simulink model "five"  (R2019b)
settings: Solver=VariableStepAuto  StartTime=0.0  StopTime=2  RelTol=1e-3
undefined symbols (not defined in the file): magnitude
libraries: dsparch4 x2, commsynccomp2 x1
settings Model: Creator=Lenovo  LastModifiedBy=Lenovo

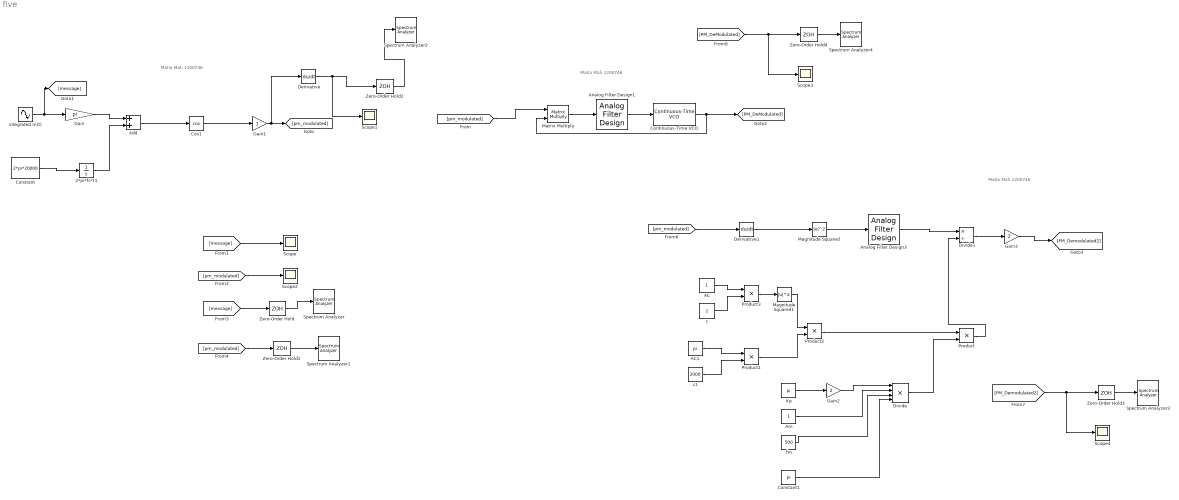
== system five ==
  note: Maha Mali 1200746
  note: Maha Mali 1200746
  note: Maha Mali 1200746
  2*pi*fc*t1 : Integrator
  AC : Constant
  AC1 : Constant  Value=pi
  Add : Sum
  Am : Constant
  Analog Filter Design1 : dsparch4/Analog Filter Design  method=Butterworth  filttype=Lowpass  N=8  Wlo=pi*2*1000  Whi=80  Rp=2  Rs=40
  Analog Filter Design3 : dsparch4/Analog Filter Design  method=Butterworth  filttype=Bandpass  N=8  Wlo=pi*2*400  Whi=pi*2*600  Rp=2  Rs=40
  Constant : Constant  Value=2*pi*20000
  Constant1 : Constant  Value=pi
  Continuous-Time VCO : commsynccomp2/Continuous-Time VCO  Ac=1  Fc=400  Kc=1  Ph=0
      settings: SourceProductName=Communications Toolbox  SourceProductBaseCode=CM
  Cos1 : Trigonometry  Operator=cos
  Derivative : Derivative
  Derivative1 : Derivative
  Divide : Product  Inputs=****
  Divide1 : Product  Inputs=*/
  Gain : Gain  Gain=pi
  Gain1 : Gain
  Gain2 : Gain  Gain=2
  Gain3 : Gain  Gain=2
  Kp : Constant  Value=pi
  Magnitude Squared : Math  Operator=magnitude^2  SignedPower=off  SaturateOnIntegerOverflow=on
  Magnitude Squared1 : Math  Operator=magnitude^2  SignedPower=off  SaturateOnIntegerOverflow=on
  Matrix Multiply : Product  Multiplication=Matrix(*)
  Product{,1..3} (4 alike) : Product
  Scope{,1..4} (5 alike) : Scope
  Spectrum Analyzer{,1..4} (5 alike) : SpectrumAnalyzer
  Zero-Order Hold : ZeroOrderHold  SampleTime=1/(10*5e2)
  Zero-Order Hold{1..4} (4 alike) : ZeroOrderHold  SampleTime=1/(10*20000)
  c : Constant  Value=2
  c1 : Constant  Value=2000
  fm : Constant  Value=500
  integrated m(t) : Sin  Frequency=500*pi*2  SampleTime=0
  wires:
  Cos1/1 -> Gain1/1
  Gain/1 -> Add/1
  integrated m(t)/1 -> [message], Gain/1
  [pm_modulated] -> Matrix Multiply/1
  2*pi*fc*t1/1 -> Add/2
  Gain1/1 -> Derivative/1, [pm_modulated]
  Constant/1 -> 2*pi*fc*t1/1
  Matrix Multiply/1 -> Analog Filter Design1/1
  [message] -> Scope/1
  Analog Filter Design1/1 -> Continuous-Time VCO/1
  Continuous-Time VCO/1 -> [PM_DeModulated], Matrix Multiply/2
  [pm_modulated] -> Scope2/1
  Add/1 -> Cos1/1
  Zero-Order Hold/1 -> Spectrum Analyzer/1
  [message] -> Zero-Order Hold/1
  [pm_modulated] -> Zero-Order Hold1/1
  Zero-Order Hold1/1 -> Spectrum Analyzer1/1
  Zero-Order Hold2/1 -> Spectrum Analyzer2/1
  Derivative/1 -> Scope1/1, Zero-Order Hold2/1
  Am/1 -> Divide/2
  AC/1 -> Product3/1
  Divide/1 -> Product/2
  Magnitude Squared/1 -> Analog Filter Design3/1
  Gain2/1 -> Divide/1
  Kp/1 -> Gain2/1
  Analog Filter Design3/1 -> Divide1/1
  Zero-Order Hold3/1 -> Spectrum Analyzer3/1
  Product3/1 -> Magnitude Squared1/1
  Product2/1 -> Product/1
  fm/1 -> Divide/3
  Derivative1/1 -> Magnitude Squared/1
  c/1 -> Product3/2
  Product/1 -> Divide1/2
  [FM_Demodulated2] -> Zero-Order Hold3/1, Scope4/1
  [pm_modulated] -> Derivative1/1
  AC1/1 -> Product1/1
  c1/1 -> Product1/2
  Product1/1 -> Product2/2
  Magnitude Squared1/1 -> Product2/1
  Constant1/1 -> Divide/4
  Divide1/1 -> Gain3/1
  Gain3/1 -> [FM_Demodulated2]
  [PM_DeModulated] -> Zero-Order Hold4/1, Scope3/1
  Zero-Order Hold4/1 -> Spectrum Analyzer4/1
